simulink model "CONTROL_02"  (R2018b)
settings: Solver=FixedStepAuto  StartTime=0.0  StopTime=10  FixedStep=0.01  RelTol=1e-3
model workspace: external: MATLAB File D:\OneDrive\STUDY\RIC LAB\PROJECT 6DOF\CODE\CODE 6DOF\07_CONTROL\CONTROL_02\ROBOT_DataFile.m (data not in the file)
values from neighbouring files (symbols this model uses):
  k1 = [k11 k12 k13 k14 k15 k16]    [GA_CTC_01.m]
  k2 = [k21 k22 k23 k24 k25 k26]    [GA_CTC_01.m]
undefined symbols (not defined in the file or in its folder): smiData, X, Y, Z
libraries: sm_lib x35, nesl_utility x7
(part 1 of 14)
settings Model: Creator=TMP  LastModifiedBy=TMP
settings DataIOCC: SaveTime=off

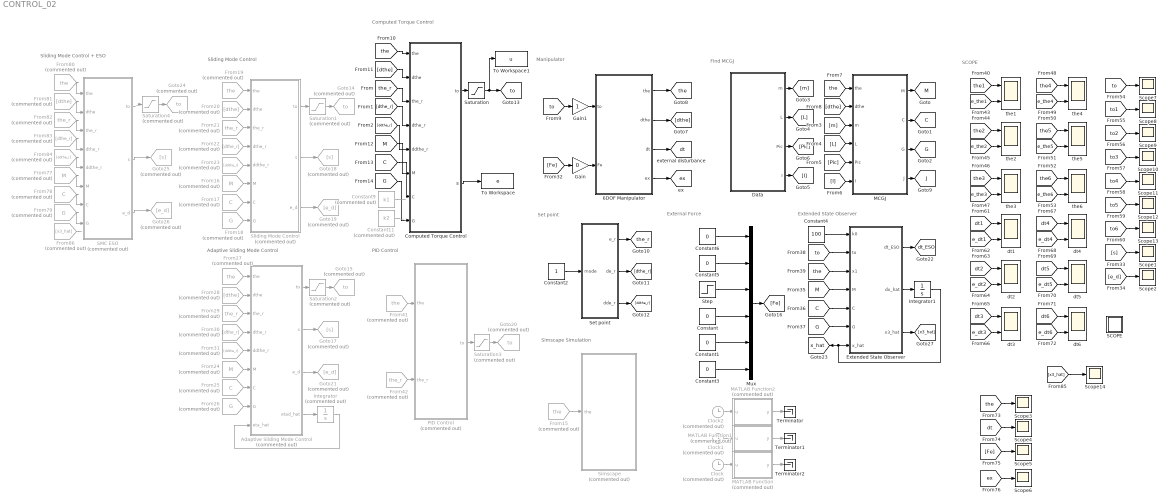
== system CONTROL_02 ==
  note: Extended State Observer
  note: SCOPE
  note: Set point
  note: Manipulator
  note: Simscape Simulation
  note: Find MCGJ
  note: Computed Torque Control
  note: Sliding Mode Control
  note: Adaptive Sliding Mode Control
  note: PID Control
  note: External Force
  note: Sliding Mode Control + ESO
  6DOF Manipulator : Subsystem
  Adaptive Sliding Mode Control : MATLAB Function  Commented=on  TreatAsAtomicUnit=on
  Clock : Clock  Commented=on
  Clock1 : Clock  Commented=on
  Clock2 : Clock  Commented=on
  Computed Torque Control : MATLAB Function  TreatAsAtomicUnit=on
  Constant{,1,3,5..6} (5 alike) : Constant  Value=0
  Constant11 : Constant  Commented=on  Value=k2
  Constant2 : Constant
  Constant4 : Constant  Value=100
  Constant9 : Constant  Commented=on  Value=k1
  Data : MATLAB Function  TreatAsAtomicUnit=on
  Extended State Observer : MATLAB Function  TreatAsAtomicUnit=on
  From{15,19,27,80} (4 alike) : From  Commented=on  GotoTag=the  TagVisibility=global
  From16 : From  Commented=on  GotoTag=M  TagVisibility=global
  From17 : From  Commented=on  GotoTag=C  TagVisibility=global
  From18 : From  Commented=on  GotoTag=G  TagVisibility=global
  From20 : From  Commented=on  GotoTag=dthe
  From21 : From  Commented=on  GotoTag=the_r  TagVisibility=global
  From22 : From  Commented=on  GotoTag=dthe_r
  From23 : From  Commented=on  GotoTag=ddthe_r
  From24 : From  Commented=on  GotoTag=M  TagVisibility=global
  From25 : From  Commented=on  GotoTag=C  TagVisibility=global
  From26 : From  Commented=on  GotoTag=G  TagVisibility=global
  From28 : From  Commented=on  GotoTag=dthe
  From29 : From  Commented=on  GotoTag=the_r  TagVisibility=global
  From30 : From  Commented=on  GotoTag=dthe_r
  From31 : From  Commented=on  GotoTag=ddthe_r
  From41 : From  Commented=on  GotoTag=the
  From42 : From  Commented=on  GotoTag=the_r
  From77 : From  Commented=on  GotoTag=M  TagVisibility=global
  From78 : From  Commented=on  GotoTag=C  TagVisibility=global
  From79 : From  Commented=on  GotoTag=G  TagVisibility=global
  From81 : From  Commented=on  GotoTag=dthe
  From82 : From  Commented=on  GotoTag=the_r  TagVisibility=global
  From83 : From  Commented=on  GotoTag=dthe_r
  From84 : From  Commented=on  GotoTag=ddthe_r
  From86 : From  Commented=on  GotoTag=x3_hat
  Gain : Gain  Gain=0
  Gain1 : Gain
  Goto{14..15,20,24} (4 alike) : Goto  Commented=on  GotoTag=to  TagVisibility=global
  Goto17 : Goto  Commented=on  GotoTag=s
  Goto18 : Goto  Commented=on  GotoTag=s
  Goto19 : Goto  Commented=on  GotoTag=e_d
  Goto21 : Goto  Commented=on  GotoTag=e_d
  Goto25 : Goto  Commented=on  GotoTag=s
  Goto26 : Goto  Commented=on  GotoTag=e_d
  Integrator : Integrator  Commented=on  InitialCondition=zeros(6)
  Integrator1 : Integrator  InitialCondition=zeros(18,1)
  MATLAB Function : MATLAB Function  Commented=on  TreatAsAtomicUnit=on
  MATLAB Function1 : MATLAB Function  Commented=on  TreatAsAtomicUnit=on
  MATLAB Function2 : MATLAB Function  Commented=on  TreatAsAtomicUnit=on
  MCGJ : MATLAB Function  TreatAsAtomicUnit=on
  Mux : Mux  Inputs=6
  PID Control : Subsystem  Commented=on
  SCOPE : Subsystem
  SMC ESO : MATLAB Function  Commented=on  TreatAsAtomicUnit=on
  Saturation : Saturate  UpperLimit=500  LowerLimit=-500
  Saturation1 : Saturate  Commented=on  UpperLimit=500  LowerLimit=-500
  Saturation2 : Saturate  Commented=on  UpperLimit=400  LowerLimit=-400
  Saturation3 : Saturate  Commented=on  UpperLimit=500  LowerLimit=-500
  Saturation4 : Saturate  Commented=on  UpperLimit=500  LowerLimit=-500
  Scope{1..14} (14 alike) : Scope
  Set point : Subsystem
  Simscape : Subsystem  Commented=on
  Sliding Mode Control : MATLAB Function  Commented=on  TreatAsAtomicUnit=on
  Step : Step  Time=5  After=20  SampleTime=0
  Terminator : Terminator
  Terminator1 : Terminator
  Terminator2 : Terminator
  To Workspace : ToWorkspace  VariableName=e  SampleTime=-1
  To Workspace1 : ToWorkspace  VariableName=u  SampleTime=-1
  dt{1..6} (6 alike) : Scope  NumInputPorts=2
  the{1..6} (6 alike) : Scope  NumInputPorts=2
  tag scope: C=global, G=global, J=global, M=global, dt=global, dt_ESO=global, ex=global, the=global, the_r=global, to=global, x_hat=global
  wires:
  [the_r] -> Computed Torque Control/3(the_r)
  Set point/3(dde_r) -> [ddthe_r]
  MCGJ/4(J) -> [J]
  [dthe] -> MCGJ/2(dthe)
  Set point/1(e_r) -> [the_r]
  [the] -> Computed Torque Control/1(the)
  [G] -> Computed Torque Control/8(G)
  [the] -> MCGJ/1(the)
  [dthe_r] -> Computed Torque Control/4(dthe_r)
  [C] -> Computed Torque Control/7(C)
  [M] -> Computed Torque Control/6(M)
  [ddthe_r] -> Computed Torque Control/5(ddthe_r)
  Constant2/1 -> Set point/1(mode)
  [m] -> MCGJ/3(m)
  Set point/2(de_r) -> [dthe_r]
  [dthe] -> Computed Torque Control/2(dthe)
  [L] -> MCGJ/4(L)
  MCGJ/3(G) -> [G]
  MCGJ/2(C) -> [C]
  [Pic] -> MCGJ/5(Pic)
  Saturation/1 -> To Workspace1/1, [to]
  [I] -> MCGJ/6(I)
  Computed Torque Control/1(to) -> Saturation/1
  MCGJ/1(M) -> [M]
  From16/1 -> Sliding Mode Control/6(M)
  From17/1 -> Sliding Mode Control/7(C)
  From18/1 -> Sliding Mode Control/8(G)
  From19/1 -> Sliding Mode Control/1(the)
  From20/1 -> Sliding Mode Control/2(dthe)
  From21/1 -> Sliding Mode Control/3(the_r)
  From22/1 -> Sliding Mode Control/4(dthe_r)
  From23/1 -> Sliding Mode Control/5(ddthe_r)
  Sliding Mode Control/1(to) -> Saturation1/1
  Saturation2/1 -> Goto15/1
  Adaptive Sliding Mode Control/1(to) -> Saturation2/1
  From31/1 -> Adaptive Sliding Mode Control/5(ddthe_r)
  From30/1 -> Adaptive Sliding Mode Control/4(dthe_r)
  From29/1 -> Adaptive Sliding Mode Control/3(the_r)
  From28/1 -> Adaptive Sliding Mode Control/2(dthe)
  From27/1 -> Adaptive Sliding Mode Control/1(the)
  From26/1 -> Adaptive Sliding Mode Control/8(G)
  From25/1 -> Adaptive Sliding Mode Control/7(C)
  From24/1 -> Adaptive Sliding Mode Control/6(M)
  Data/1(m) -> [m]
  Data/2(L) -> [L]
  Data/3(Pic) -> [Pic]
  Data/4(I) -> [I]
  6DOF Manipulator/2(dthe) -> [dthe]
  6DOF Manipulator/1(the) -> [the]
  From15/1 -> Simscape/1(the)
  Saturation1/1 -> Goto14/1
  [Fe] -> Gain/1
  Gain/1 -> 6DOF Manipulator/2(Fe)
  Adaptive Sliding Mode Control/2(s) -> Goto17/1
  Sliding Mode Control/2(s) -> Goto18/1
  Constant1/1 -> Mux/5
  Mux/1 -> [Fe]
  Constant3/1 -> Mux/6
  Constant/1 -> Mux/4
  PID Control/1(to) -> Saturation3/1
  From41/1 -> PID Control/1(the)
  From42/1 -> PID Control/2(the_r)
  Saturation3/1 -> Goto20/1
  6DOF Manipulator/3(dt) -> [dt]
  [to] -> Gain1/1
  Gain1/1 -> 6DOF Manipulator/1(to)
  Sliding Mode Control/3(e_d) -> Goto19/1
  Adaptive Sliding Mode Control/3(e_d) -> Goto21/1
  [the1] -> the1/1
  [e_the1] -> the1/2
  [e_the2] -> the2/2
  [the2] -> the2/1
  [the3] -> the3/1
  [e_the3] -> the3/2
  [e_the6] -> the6/2
  [the6] -> the6/1
  [the5] -> the5/1
  [e_the5] -> the5/2
  [e_the4] -> the4/2
  [the4] -> the4/1
  [to] -> Scope7/1
  [to1] -> Scope8/1
  [to2] -> Scope9/1
  [to5] -> Scope12/1
  [to4] -> Scope11/1
  [to3] -> Scope10/1
  [to6] -> Scope13/1
  [s] -> Scope1/1
  [e_d] -> Scope2/1
  Adaptive Sliding Mode Control/4(etad_hat) -> Integrator/1
  Integrator/1 -> Adaptive Sliding Mode Control/9(eta_hat)
  Extended State Observer/1(dt_ESO) -> [dt_ESO]
  Extended State Observer/2(dx_hat) -> Integrator1/1
  Constant4/1 -> Extended State Observer/1(k0)
  [to] -> Extended State Observer/2(to)
  [the] -> Extended State Observer/3(x1)
  [M] -> Extended State Observer/4(M)
  [C] -> Extended State Observer/5(C)
  [G] -> Extended State Observer/6(G)
  Integrator1/1 -> [x_hat], Extended State Observer/7(x_hat)
  [dt4] -> dt4/1
  [e_dt4] -> dt4/2
  [e_dt5] -> dt5/2
  [dt5] -> dt5/1
  [dt6] -> dt6/1
  [e_dt6] -> dt6/2
  [e_dt3] -> dt3/2
  [dt3] -> dt3/1
  [dt2] -> dt2/1
  [e_dt2] -> dt2/2
  [e_dt1] -> dt1/2
  [dt1] -> dt1/1
  [the] -> Scope3/1
  [dt] -> Scope4/1
  MATLAB Function1/1(y) -> Terminator1/1
  Clock1/1 -> MATLAB Function1/1(u)
  Clock/1 -> MATLAB Function/1(u)
  MATLAB Function/1(y) -> Terminator2/1
  Clock2/1 -> MATLAB Function2/1(u)
  MATLAB Function2/1(y) -> Terminator/1
  Step/1 -> Mux/3
  Constant6/1 -> Mux/1
  Constant5/1 -> Mux/2
  [Fe] -> Scope5/1
  6DOF Manipulator/4(ex) -> [ex]
  [ex] -> Scope6/1
  Computed Torque Control/2(E) -> To Workspace/1
  Constant9/1 -> ?
  Constant11/1 -> ?
  SMC ESO/3(e_d) -> Goto26/1
  SMC ESO/2(s) -> Goto25/1
  Saturation4/1 -> Goto24/1
  SMC ESO/1(to) -> Saturation4/1
  From84/1 -> SMC ESO/5(ddthe_r)
  From83/1 -> SMC ESO/4(dthe_r)
  From82/1 -> SMC ESO/3(the_r)
  From81/1 -> SMC ESO/2(dthe)
  From80/1 -> SMC ESO/1(the)
  From79/1 -> SMC ESO/8(G)
  From78/1 -> SMC ESO/7(C)
  From77/1 -> SMC ESO/6(M)
  From86/1 -> ?
  Extended State Observer/3(x3_hat) -> [x3_hat]
  [x3_hat] -> Scope14/1

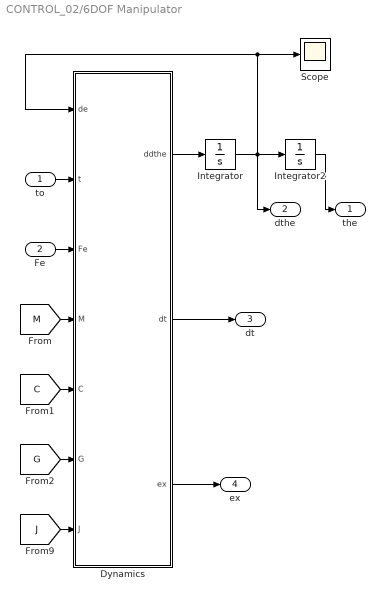
== system CONTROL_02/6DOF Manipulator ==
  to : Inport
  Fe : Inport  Port=2
  Dynamics : MATLAB Function  TreatAsAtomicUnit=on
  Integrator : Integrator  InitialCondition=[0;0;0;0;0;0]  UpperSaturationLimit=pi  LowerSaturationLimit=-pi
  Integrator2 : Integrator  InitialCondition=[0;0;0;0;0;0]  UpperSaturationLimit=[170;135;166;190;120;360]*pi/180  LowerSaturationLimit=-[170;100;119;190;120;360]*pi/180
  Scope : Scope
  the : Outport
  dthe : Outport  Port=2
  dt : Outport  Port=3
  ex : Outport  Port=4
  wires:
  Integrator2/1 -> the/1
  Dynamics/1(ddthe) -> Integrator/1
  [C] -> Dynamics/5(C)
  [J] -> Dynamics/7(J)
  Integrator/1 -> Integrator2/1, Scope/1, Dynamics/1(de), dthe/1
  [M] -> Dynamics/4(M)
  [G] -> Dynamics/6(G)
  to/1 -> Dynamics/2(t)
  Dynamics/2(dt) -> dt/1
  Fe/1 -> Dynamics/3(Fe)
  Dynamics/3(ex) -> ex/1

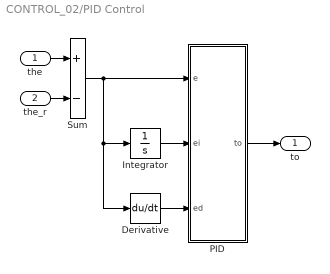
== system CONTROL_02/PID Control ==
  the : Inport
  the_r : Inport  Port=2
  Derivative : Derivative
  Integrator : Integrator
  PID : MATLAB Function  TreatAsAtomicUnit=on
  Sum : Sum  Inputs=+-
  to : Outport
  wires:
  Sum/1 -> Derivative/1, Integrator/1, PID/1(e)
  the/1 -> Sum/1
  the_r/1 -> Sum/2
  PID/1(to) -> to/1
  Derivative/1 -> PID/3(ed)
  Integrator/1 -> PID/2(ei)

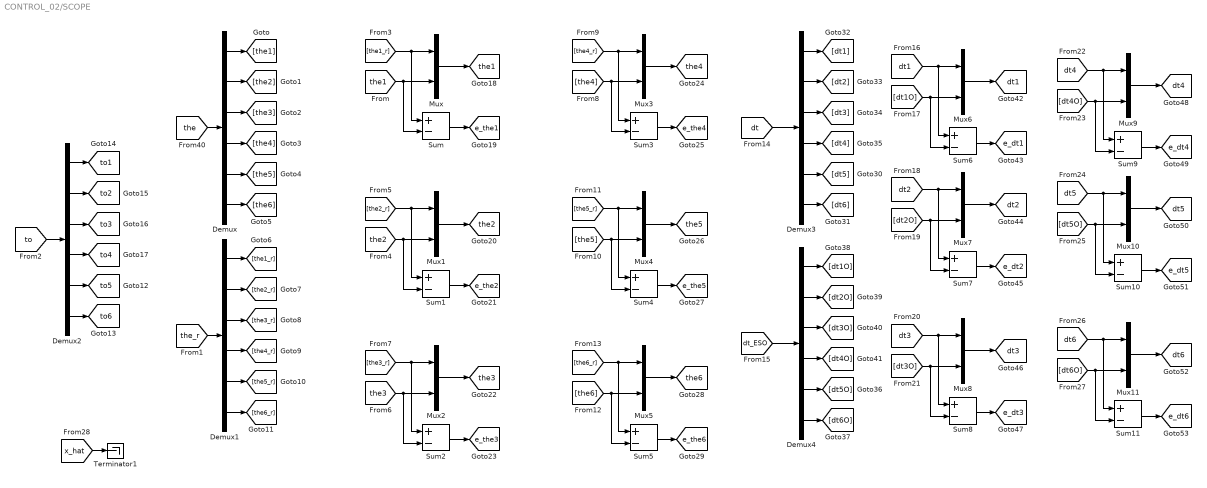
== system CONTROL_02/SCOPE ==
  Demux{,1..4} (5 alike) : Demux  Outputs=6
  Mux{,1..11} (12 alike) : Mux  Inputs=2
  Sum{,1..11} (12 alike) : Sum  Inputs=+-
  Terminator1 : Terminator
  tag scope: dt1=global, dt2=global, dt3=global, dt4=global, dt5=global, dt6=global, e_dt1=global, e_dt2=global, e_dt3=global, e_dt4=global, e_dt5=global, e_dt6=global, e_the1=global, e_the2=global, e_the3=global, e_the4=global, e_the5=global, e_the6=global, the1=global, the2=global, the3=global, the4=global, the5=global, the6=global, to1=global, to2=global, to3=global, to4=global, to5=global, to6=global
  wires:
  Demux/4 -> [the4]
  Demux/6 -> [the6]
  [the] -> Demux/1
  Demux/1 -> [the1]
  Demux/5 -> [the5]
  Demux/2 -> [the2]
  Demux/3 -> [the3]
  Demux1/1 -> [the1_r]
  Demux1/4 -> [the4_r]
  [the_r] -> Demux1/1
  Demux1/5 -> [the5_r]
  Demux1/2 -> [the2_r]
  Demux1/3 -> [the3_r]
  Demux1/6 -> [the6_r]
  Demux2/6 -> [to6]
  Demux2/3 -> [to3]
  Demux2/2 -> [to2]
  Demux2/4 -> [to4]
  Demux2/5 -> [to5]
  [to] -> Demux2/1
  Demux2/1 -> [to1]
  [the1_r] -> Sum/1, Mux/1
  [the1] -> Mux/2, Sum/2
  Mux/1 -> [the1]
  Sum/1 -> [e_the1]
  Sum1/1 -> [e_the2]
  Mux1/1 -> [the2]
  [the2] -> Sum1/2, Mux1/2
  [the2_r] -> Mux1/1, Sum1/1
  [the3_r] -> Sum2/1, Mux2/1
  [the3] -> Mux2/2, Sum2/2
  Mux2/1 -> [the3]
  Sum2/1 -> [e_the3]
  Sum5/1 -> [e_the6]
  Mux5/1 -> [the6]
  [the6] -> Sum5/2, Mux5/2
  [the6_r] -> Mux5/1, Sum5/1
  [the5_r] -> Sum4/1, Mux4/1
  [the5] -> Mux4/2, Sum4/2
  Mux4/1 -> [the5]
  Sum4/1 -> [e_the5]
  Sum3/1 -> [e_the4]
  Mux3/1 -> [the4]
  [the4] -> Sum3/2, Mux3/2
  [the4_r] -> Mux3/1, Sum3/1
  Demux3/1 -> [dt1]
  Demux3/5 -> [dt5]
  Demux3/4 -> [dt4]
  Demux3/2 -> [dt2]
  Demux3/3 -> [dt3]
  Demux3/6 -> [dt6]
  [dt] -> Demux3/1
  [dt_ESO] -> Demux4/1
  Demux4/6 -> [dt6O]
  Demux4/3 -> [dt3O]
  Demux4/2 -> [dt2O]
  Demux4/4 -> [dt4O]
  Demux4/5 -> [dt5O]
  Demux4/1 -> [dt1O]
  Sum6/1 -> [e_dt1]
  Mux6/1 -> [dt1]
  [dt1O] -> Sum6/2, Mux6/2
  [dt1] -> Mux6/1, Sum6/1
  [dt2] -> Sum7/1, Mux7/1
  [dt2O] -> Mux7/2, Sum7/2
  Mux7/1 -> [dt2]
  Sum7/1 -> [e_dt2]
  Sum8/1 -> [e_dt3]
  Mux8/1 -> [dt3]
  [dt3O] -> Sum8/2, Mux8/2
  [dt3] -> Mux8/1, Sum8/1
  [dt6] -> Sum11/1, Mux11/1
  [dt6O] -> Mux11/2, Sum11/2
  Mux11/1 -> [dt6]
  Sum11/1 -> [e_dt6]
  Sum10/1 -> [e_dt5]
  Mux10/1 -> [dt5]
  [dt5O] -> Sum10/2, Mux10/2
  [dt5] -> Mux10/1, Sum10/1
  [dt4] -> Sum9/1, Mux9/1
  [dt4O] -> Mux9/2, Sum9/2
  Mux9/1 -> [dt4]
  Sum9/1 -> [e_dt4]
  [x_hat] -> Terminator1/1

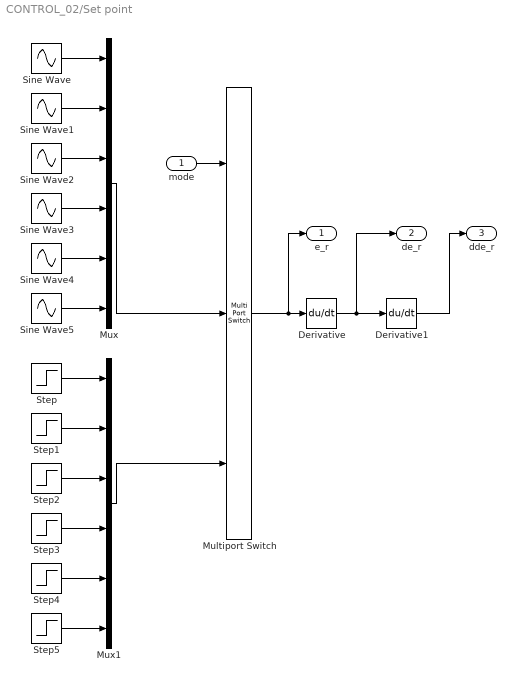
== system CONTROL_02/Set point ==
  mode : Inport
  Derivative : Derivative
  Derivative1 : Derivative
  Multiport Switch : MultiPortSwitch  Inputs=2
  Mux : Mux  Inputs=6
  Mux1 : Mux  Inputs=6
  Sine Wave{,1..5} (6 alike) : Sin  Amplitude=pi/6  Frequency=2*pi*0.1  SampleTime=0
  Step{,1..5} (6 alike) : Step  After=0  SampleTime=0
  e_r : Outport
  de_r : Outport  Port=2
  dde_r : Outport  Port=3
  wires:
  Sine Wave/1 -> Mux/1
  Sine Wave1/1 -> Mux/2
  Sine Wave2/1 -> Mux/3
  Sine Wave3/1 -> Mux/4
  Sine Wave4/1 -> Mux/5
  Sine Wave5/1 -> Mux/6
  Mux/1 -> Multiport Switch/2
  Mux1/1 -> Multiport Switch/3
  Step2/1 -> Mux1/3
  Step5/1 -> Mux1/6
  Step1/1 -> Mux1/2
  Step3/1 -> Mux1/4
  Step/1 -> Mux1/1
  Step4/1 -> Mux1/5
  Multiport Switch/1 -> e_r/1, Derivative/1
  Derivative/1 -> de_r/1, Derivative1/1
  Derivative1/1 -> dde_r/1
  mode/1 -> Multiport Switch/1

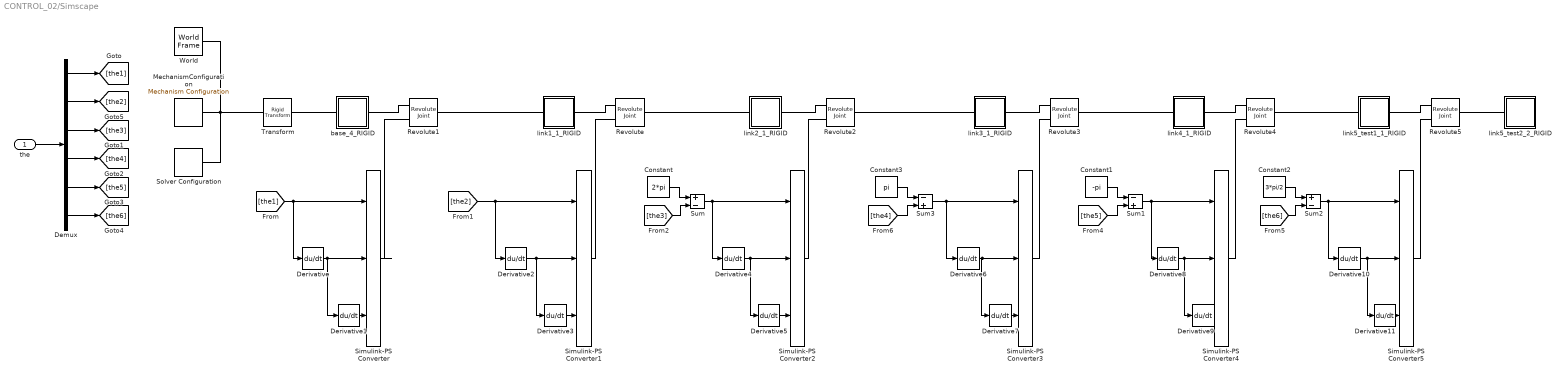
== system CONTROL_02/Simscape ==
  the : Inport
  Constant : Constant  Value=2*pi
  Constant1 : Constant  Value=-pi
  Constant2 : Constant  Value=3*pi/2
  Constant3 : Constant  Value=pi
  Demux : Demux  Outputs=6
  Derivative{,1..11} (12 alike) : Derivative
  MechanismConfiguration : sm_lib/Utilities/Mechanism Configuration  UniformGravity=Constant  GravityVector=[0 -9.80665 0]  GravityUnits=m/s^2  LinearizationDelta=0.001
  Revolute : sm_lib/Joints/Revolute Joint  SenseConstraintForce=off  SenseConstraintForceX=off  SenseConstraintForceY=off  SenseConstraintForceZ=off  SenseConstraintTorque=off  SenseConstraintTorqueX=off  SenseConstraintTorqueY=off  SenseConstraintTorqueZ=off  SenseTotalForce=off  SenseTotalForceX=off  SenseTotalForceY=off  SenseTotalForceZ=off  SenseTotalTorque=off  SenseTotalTorqueX=off  SenseTotalTorqueY=off  SenseTotalTorqueZ=off  CompositeWrenchDir=FollowerOnBase  CompositeWrenchFrame=BaseFrame  EquilibriumPosition=0  EquilibriumPositionUnits=rad  SpringStiffness=0  SpringStiffnessUnits=N*m/rad  DampingCoefficient=0  DampingCoefficientUnits=N*m/(rad/s)  TorqueActuationMode=ComputedTorque  MotionActuationMode=InputMotion  SensePosition=off  SenseVelocity=off  SenseAcceleration=off  SenseTorqueForce=off  PositionTargetSpecify=on  PositionTargetPriority=Low  PositionTargetValue=smiData.RevoluteJoint(1).Rz.Pos  PositionTargetValueUnits=deg  VelocityTargetSpecify=off  VelocityTargetPriority=High  VelocityTargetValue=0  VelocityTargetValueUnits=deg/s
  Revolute1 : sm_lib/Joints/Revolute Joint  SenseConstraintForce=off  SenseConstraintForceX=off  SenseConstraintForceY=off  SenseConstraintForceZ=off  SenseConstraintTorque=off  SenseConstraintTorqueX=off  SenseConstraintTorqueY=off  SenseConstraintTorqueZ=off  SenseTotalForce=off  SenseTotalForceX=off  SenseTotalForceY=off  SenseTotalForceZ=off  SenseTotalTorque=off  SenseTotalTorqueX=off  SenseTotalTorqueY=off  SenseTotalTorqueZ=off  CompositeWrenchDir=FollowerOnBase  CompositeWrenchFrame=BaseFrame  EquilibriumPosition=0  EquilibriumPositionUnits=rad  SpringStiffness=0  SpringStiffnessUnits=N*m/rad  DampingCoefficient=0  DampingCoefficientUnits=N*m/(rad/s)  TorqueActuationMode=ComputedTorque  MotionActuationMode=InputMotion  SensePosition=off  SenseVelocity=off  SenseAcceleration=off  SenseTorqueForce=off  PositionTargetSpecify=on  PositionTargetPriority=Low  PositionTargetValue=smiData.RevoluteJoint(2).Rz.Pos  PositionTargetValueUnits=deg  VelocityTargetSpecify=off  VelocityTargetPriority=High  VelocityTargetValue=0  VelocityTargetValueUnits=deg/s
  Revolute2 : sm_lib/Joints/Revolute Joint  SenseConstraintForce=off  SenseConstraintForceX=off  SenseConstraintForceY=off  SenseConstraintForceZ=off  SenseConstraintTorque=off  SenseConstraintTorqueX=off  SenseConstraintTorqueY=off  SenseConstraintTorqueZ=off  SenseTotalForce=off  SenseTotalForceX=off  SenseTotalForceY=off  SenseTotalForceZ=off  SenseTotalTorque=off  SenseTotalTorqueX=off  SenseTotalTorqueY=off  SenseTotalTorqueZ=off  CompositeWrenchDir=FollowerOnBase  CompositeWrenchFrame=BaseFrame  EquilibriumPosition=0  EquilibriumPositionUnits=rad  SpringStiffness=0  SpringStiffnessUnits=N*m/rad  DampingCoefficient=0  DampingCoefficientUnits=N*m/(rad/s)  TorqueActuationMode=ComputedTorque  MotionActuationMode=InputMotion  SensePosition=off  SenseVelocity=off  SenseAcceleration=off  SenseTorqueForce=off  PositionTargetSpecify=on  PositionTargetPriority=Low  PositionTargetValue=smiData.RevoluteJoint(3).Rz.Pos  PositionTargetValueUnits=deg  VelocityTargetSpecify=off  VelocityTargetPriority=High  VelocityTargetValue=0  VelocityTargetValueUnits=deg/s
  Revolute3 : sm_lib/Joints/Revolute Joint  SenseConstraintForce=off  SenseConstraintForceX=off  SenseConstraintForceY=off  SenseConstraintForceZ=off  SenseConstraintTorque=off  SenseConstraintTorqueX=off  SenseConstraintTorqueY=off  SenseConstraintTorqueZ=off  SenseTotalForce=off  SenseTotalForceX=off  SenseTotalForceY=off  SenseTotalForceZ=off  SenseTotalTorque=off  SenseTotalTorqueX=off  SenseTotalTorqueY=off  SenseTotalTorqueZ=off  CompositeWrenchDir=FollowerOnBase  CompositeWrenchFrame=BaseFrame  EquilibriumPosition=0  EquilibriumPositionUnits=rad  SpringStiffness=0  SpringStiffnessUnits=N*m/rad  DampingCoefficient=0  DampingCoefficientUnits=N*m/(rad/s)  TorqueActuationMode=ComputedTorque  MotionActuationMode=InputMotion  SensePosition=off  SenseVelocity=off  SenseAcceleration=off  SenseTorqueForce=off  PositionTargetSpecify=on  PositionTargetPriority=Low  PositionTargetValue=smiData.RevoluteJoint(4).Rz.Pos  PositionTargetValueUnits=deg  VelocityTargetSpecify=off  VelocityTargetPriority=High  VelocityTargetValue=0  VelocityTargetValueUnits=deg/s
  Revolute4 : sm_lib/Joints/Revolute Joint  SenseConstraintForce=off  SenseConstraintForceX=off  SenseConstraintForceY=off  SenseConstraintForceZ=off  SenseConstraintTorque=off  SenseConstraintTorqueX=off  SenseConstraintTorqueY=off  SenseConstraintTorqueZ=off  SenseTotalForce=off  SenseTotalForceX=off  SenseTotalForceY=off  SenseTotalForceZ=off  SenseTotalTorque=off  SenseTotalTorqueX=off  SenseTotalTorqueY=off  SenseTotalTorqueZ=off  CompositeWrenchDir=FollowerOnBase  CompositeWrenchFrame=BaseFrame  EquilibriumPosition=0  EquilibriumPositionUnits=rad  SpringStiffness=0  SpringStiffnessUnits=N*m/rad  DampingCoefficient=0  DampingCoefficientUnits=N*m/(rad/s)  TorqueActuationMode=ComputedTorque  MotionActuationMode=InputMotion  SensePosition=off  SenseVelocity=off  SenseAcceleration=off  SenseTorqueForce=off  PositionTargetSpecify=on  PositionTargetPriority=Low  PositionTargetValue=smiData.RevoluteJoint(5).Rz.Pos  PositionTargetValueUnits=deg  VelocityTargetSpecify=off  VelocityTargetPriority=High  VelocityTargetValue=0  VelocityTargetValueUnits=deg/s
  Revolute5 : sm_lib/Joints/Revolute Joint  SenseConstraintForce=off  SenseConstraintForceX=off  SenseConstraintForceY=off  SenseConstraintForceZ=off  SenseConstraintTorque=off  SenseConstraintTorqueX=off  SenseConstraintTorqueY=off  SenseConstraintTorqueZ=off  SenseTotalForce=off  SenseTotalForceX=off  SenseTotalForceY=off  SenseTotalForceZ=off  SenseTotalTorque=off  SenseTotalTorqueX=off  SenseTotalTorqueY=off  SenseTotalTorqueZ=off  CompositeWrenchDir=FollowerOnBase  CompositeWrenchFrame=BaseFrame  EquilibriumPosition=0  EquilibriumPositionUnits=rad  SpringStiffness=0  SpringStiffnessUnits=N*m/rad  DampingCoefficient=0  DampingCoefficientUnits=N*m/(rad/s)  TorqueActuationMode=ComputedTorque  MotionActuationMode=InputMotion  SensePosition=off  SenseVelocity=off  SenseAcceleration=off  SenseTorqueForce=off  PositionTargetSpecify=on  PositionTargetPriority=Low  PositionTargetValue=smiData.RevoluteJoint(6).Rz.Pos  PositionTargetValueUnits=deg  VelocityTargetSpecify=off  VelocityTargetPriority=High  VelocityTargetValue=0  VelocityTargetValueUnits=deg/s
  Simulink-PS Converter{,1..5} (6 alike) : nesl_utility/Simulink-PS Converter  PhysicalDomain=network_engine_domain  SubClassName=ps_input  LeftPortType=input  RightPortType=output  PseudoPeriodic=off  Frequencies=[]  NoiseDistribution=none  NoiseParameters=[]  Unit=1  AffineConversion=off  FilteringAndDerivatives=provide  SimscapeFilterOrder=1  InputFilterTimeConstant=0.001  UdotUserProvided=2
  Solver Configuration : nesl_utility/Solver Configuration  PhysicalDomain=network_engine_domain  SubClassName=solver  LeftPortType=input  RightPortType=generic  Tones=[]  Harmonics=[]  SimulateNoise=off  Profile=off  UseLocalSampling=off  EnableSwitchedLinearOptims=on  FrequencyDomain=off  UseCCode=off  RelTol=0.001  AbsTol=1e-06  MinStep=1e-09  ToWorkspace=off  RevertToSquareIcSolve=off  NumHomotopyIterations=100  PhasorMode=off  PhasorModeNumHarmonics=1  DoDC=off  ResidualTolerance=1e-09  UseLocalSolver=off  LocalSolverChoice=NE_BACKWARD_EULER_ADVANCER  LocalSolverSampleTime=0.001  DoFixedCost=off  MaxNonlinIter=3  MaxModeIter=2  LinearAlgebra=auto  EquationFormulation=NE_TIME_EF  DelaysMemoryBudget=1024  AutomaticFiltering=on  FilteringTimeConstant=0.001  PartitionStorageMethod=AS_NEEDED  PartitionMemoryBudget=1024
  Sum : Sum  Inputs=+-
  Sum1 : Sum  Inputs=-+
  Sum2 : Sum  Inputs=+-
  Sum3 : Sum  Inputs=-+
  Transform : sm_lib/Frames and Transforms/Rigid Transform  TranslationMethod=Cartesian  TranslationStandardOffset=0  TranslationLengthUnit=m  TranslationStandardAxis=+Z  TranslationCartesianOffset=smiData.RigidTransform(13).translation  TranslationROffset=0  TranslationROffsetUnits=m  TranslationZOffset=0  TranslationZOffsetUnits=m  TranslationThetaOffset=0  TranslationThetaOffsetUnits=deg  RotationMethod=ArbitraryAxis  RotationAngleUnits=rad  RotationStandardAxis=+Z  RotationAngle=smiData.RigidTransform(13).angle  RotationArbitraryAxis=smiData.RigidTransform(13).axis  FollAlignAxisA=+X  BaseAlignAxisA=+Y  FollAlignAxisB=+Y  BaseAlignAxisB=+Z  RotationSequenceAxes=FollowerAxes  RotationSequence=XYX  RotationSequenceAngles=[0 0 0]  RotationSequenceAnglesUnits=deg  RotationMatrix=[1 0 0; 0 1 0; 0 0 1]
  World : sm_lib/Frames and Transforms/World Frame
  base_4_RIGID : Subsystem
  link1_1_RIGID : Subsystem
  link2_1_RIGID : Subsystem
  link3_1_RIGID : Subsystem
  link4_1_RIGID : Subsystem
  link5_test1_1_RIGID : Subsystem
  link5_test2_2_RIGID : Subsystem
  wires:
  Derivative2/1 -> Derivative3/1, Simulink-PS Converter1/2
  [the2] -> Derivative2/1, Simulink-PS Converter1/1
  Derivative11/1 -> Simulink-PS Converter5/3
  [the6] -> Sum2/2
  Demux/5 -> [the5]
  Sum3/1 -> Derivative6/1, Simulink-PS Converter3/1
  [the3] -> Sum/2
  Derivative4/1 -> Derivative5/1, Simulink-PS Converter2/2
  Derivative7/1 -> Simulink-PS Converter3/3
  Demux/1 -> [the1]
  Sum/1 -> Simulink-PS Converter2/1, Derivative4/1
  Sum1/1 -> Derivative8/1, Simulink-PS Converter4/1
  Derivative8/1 -> Derivative9/1, Simulink-PS Converter4/2
  Demux/2 -> [the2]
  Demux/3 -> [the3]
  Derivative10/1 -> Simulink-PS Converter5/2, Derivative11/1
  Demux/4 -> [the4]
  the/1 -> Demux/1
  [the5] -> Sum1/2
  Demux/6 -> [the6]
  Sum2/1 -> Derivative10/1, Simulink-PS Converter5/1
  [the1] -> Derivative/1, Simulink-PS Converter/1
  Derivative6/1 -> Derivative7/1, Simulink-PS Converter3/2
  Constant2/1 -> Sum2/1
  Derivative/1 -> Derivative1/1, Simulink-PS Converter/2
  Derivative5/1 -> Simulink-PS Converter2/3
  Derivative1/1 -> Simulink-PS Converter/3
  Constant1/1 -> Sum1/1
  Derivative9/1 -> Simulink-PS Converter4/3
  Derivative3/1 -> Simulink-PS Converter1/3
  Constant/1 -> Sum/1
  Constant3/1 -> Sum3/1
  [the4] -> Sum3/2
  connections:
  Simulink-PS Converter/RConn1 -- Revolute1/LConn2
  Revolute/RConn1 -- link2_1_RIGID/LConn1
  Revolute3/RConn1 -- link4_1_RIGID/LConn1
  Revolute1/RConn1 -- link1_1_RIGID/LConn1
  Revolute4/LConn2 -- Simulink-PS Converter4/RConn1
  Revolute2/LConn2 -- Simulink-PS Converter2/RConn1
  Transform/RConn1 -- base_4_RIGID/LConn1
  Revolute1/LConn1 -- base_4_RIGID/RConn1
  Revolute/LConn1 -- link1_1_RIGID/RConn1
  Revolute/LConn2 -- Simulink-PS Converter1/RConn1
  Revolute4/RConn1 -- link5_test1_1_RIGID/LConn1
  Revolute5/LConn1 -- link5_test1_1_RIGID/RConn1
  Revolute3/LConn2 -- Simulink-PS Converter3/RConn1
  Revolute5/RConn1 -- link5_test2_2_RIGID/LConn1
  Transform/LConn1 -- MechanismConfiguration/RConn1 -- Solver Configuration/RConn1 -- World/RConn1
  Revolute5/LConn2 -- Simulink-PS Converter5/RConn1
  Revolute2/RConn1 -- link3_1_RIGID/LConn1
  Revolute2/LConn1 -- link2_1_RIGID/RConn1
  Revolute3/LConn1 -- link3_1_RIGID/RConn1
  Revolute4/LConn1 -- link4_1_RIGID/RConn1

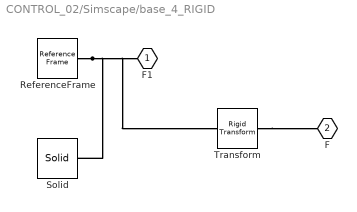
== system CONTROL_02/Simscape/base_4_RIGID ==
  ReferenceFrame : sm_lib/Frames and Transforms/Reference Frame
  Solid : sm_lib/Body Elements/Solid  InertiaType=Custom  Mass=smiData.Solid(1).mass  MassUnits=kg  CenterOfMass=smiData.Solid(1).CoM  CenterOfMassUnits=m  MomentsOfInertia=smiData.Solid(1).MoI  MomentsOfInertiaUnits=kg*m^2  ProductsOfInertia=smiData.Solid(1).PoI  ProductsOfInertiaUnits=kg*m^2  BasedOnType=Density  Density=1000  DensityUnits=kg/m^3  DoExposeReferenceFrame=on  SerializedFrames=<Frames/>  GraphicType=FromGeometry  MarkerShape=Sphere  MarkerSize=10  GraphicVisPropType=SimpleVisualProperties  GraphicDiffuseColor=smiData.Solid(1).color  GraphicSpecularColor=[0.5 0.5 0.5 1.0]  GraphicAmbientColor=[0.15 0.15 0.15 1.0]  GraphicEmissiveColor=[0.0 0.0 0.0 1.0]  GraphicShininess=75  GraphicOpacity=smiData.Solid(1).opacity  GeometryShape=FromFile  RectangleSize=[1 1]  RectangleSizeUnits=m  BrickDimensions=[1 1 1]  BrickDimensionUnits=m  CylinderRadius=1  CylinderRadiusUnits=m  CylinderLength=1  CylinderLengthUnits=m  SphereRadius=1  SphereRadiusUnits=m  EllipsoidRadii=[1 1 1]  EllipsoidRadiiUnits=m  ExtrusionCrossSection=[1 1; -1 1; -1 -1; 1 -1]  ExtrusionCrossSectionUnits=m  ExtrusionLength=1  ExtrusionLengthUnits=m  PolygonNumSides=3  PolygonOuterRadius=1  PolygonOuterRadiusUnits=m  ExtGeomFileType=STEP  ExtGeomFileName=base_Default_sldprt.STEP  ExtGeomFileUnits=m  RevolutionCrossSection=[1 1; 1 -1; 2 -1; 2 1]  RevolutionCrossSectionUnits=m  RevolutionExtent=Full  RevolutionAngle=180  RevolutionAngleUnits=deg
  Transform : sm_lib/Frames and Transforms/Rigid Transform  TranslationMethod=Cartesian  TranslationStandardOffset=0  TranslationLengthUnit=m  TranslationStandardAxis=+Z  TranslationCartesianOffset=smiData.RigidTransform(3).translation  TranslationROffset=0  TranslationROffsetUnits=m  TranslationZOffset=0  TranslationZOffsetUnits=m  TranslationThetaOffset=0  TranslationThetaOffsetUnits=deg  RotationMethod=ArbitraryAxis  RotationAngleUnits=rad  RotationStandardAxis=+Z  RotationAngle=smiData.RigidTransform(3).angle  RotationArbitraryAxis=smiData.RigidTransform(3).axis  FollAlignAxisA=+X  BaseAlignAxisA=+Y  FollAlignAxisB=+Y  BaseAlignAxisB=+Z  RotationSequenceAxes=FollowerAxes  RotationSequence=XYX  RotationSequenceAngles=[0 0 0]  RotationSequenceAnglesUnits=deg  RotationMatrix=[1 0 0; 0 1 0; 0 0 1]
  F1 : PMIOPort  Side=Left
  F : PMIOPort  Port=2  Side=Right
  connections:
  Solid/RConn1 -- ReferenceFrame/RConn1 -- Transform/LConn1 -- F1/RConn1
  Transform/RConn1 -- F/RConn1

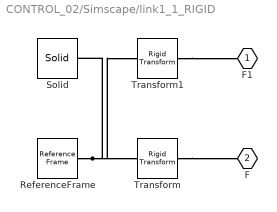
== system CONTROL_02/Simscape/link1_1_RIGID ==
  ReferenceFrame : sm_lib/Frames and Transforms/Reference Frame
  Solid : sm_lib/Body Elements/Solid  InertiaType=Custom  Mass=smiData.Solid(2).mass  MassUnits=kg  CenterOfMass=smiData.Solid(2).CoM  CenterOfMassUnits=m  MomentsOfInertia=smiData.Solid(2).MoI  MomentsOfInertiaUnits=kg*m^2  ProductsOfInertia=smiData.Solid(2).PoI  ProductsOfInertiaUnits=kg*m^2  BasedOnType=Density  Density=1000  DensityUnits=kg/m^3  DoExposeReferenceFrame=on  SerializedFrames=<Frames/>  GraphicType=FromGeometry  MarkerShape=Sphere  MarkerSize=10  GraphicVisPropType=SimpleVisualProperties  GraphicDiffuseColor=smiData.Solid(2).color  GraphicSpecularColor=[0.5 0.5 0.5 1.0]  GraphicAmbientColor=[0.15 0.15 0.15 1.0]  GraphicEmissiveColor=[0.0 0.0 0.0 1.0]  GraphicShininess=75  GraphicOpacity=smiData.Solid(2).opacity  GeometryShape=FromFile  RectangleSize=[1 1]  RectangleSizeUnits=m  BrickDimensions=[1 1 1]  BrickDimensionUnits=m  CylinderRadius=1  CylinderRadiusUnits=m  CylinderLength=1  CylinderLengthUnits=m  SphereRadius=1  SphereRadiusUnits=m  EllipsoidRadii=[1 1 1]  EllipsoidRadiiUnits=m  ExtrusionCrossSection=[1 1; -1 1; -1 -1; 1 -1]  ExtrusionCrossSectionUnits=m  ExtrusionLength=1  ExtrusionLengthUnits=m  PolygonNumSides=3  PolygonOuterRadius=1  PolygonOuterRadiusUnits=m  ExtGeomFileType=STEP  ExtGeomFileName=link1_Default_sldprt.STEP  ExtGeomFileUnits=m  RevolutionCrossSection=[1 1; 1 -1; 2 -1; 2 1]  RevolutionCrossSectionUnits=m  RevolutionExtent=Full  RevolutionAngle=180  RevolutionAngleUnits=deg
  Transform : sm_lib/Frames and Transforms/Rigid Transform  TranslationMethod=Cartesian  TranslationStandardOffset=0  TranslationLengthUnit=m  TranslationStandardAxis=+Z  TranslationCartesianOffset=smiData.RigidTransform(1).translation  TranslationROffset=0  TranslationROffsetUnits=m  TranslationZOffset=0  TranslationZOffsetUnits=m  TranslationThetaOffset=0  TranslationThetaOffsetUnits=deg  RotationMethod=ArbitraryAxis  RotationAngleUnits=rad  RotationStandardAxis=+Z  RotationAngle=smiData.RigidTransform(1).angle  RotationArbitraryAxis=smiData.RigidTransform(1).axis  FollAlignAxisA=+X  BaseAlignAxisA=+Y  FollAlignAxisB=+Y  BaseAlignAxisB=+Z  RotationSequenceAxes=FollowerAxes  RotationSequence=XYX  RotationSequenceAngles=[0 0 0]  RotationSequenceAnglesUnits=deg  RotationMatrix=[1 0 0; 0 1 0; 0 0 1]
  Transform1 : sm_lib/Frames and Transforms/Rigid Transform  TranslationMethod=Cartesian  TranslationStandardOffset=0  TranslationLengthUnit=m  TranslationStandardAxis=+Z  TranslationCartesianOffset=smiData.RigidTransform(4).translation  TranslationROffset=0  TranslationROffsetUnits=m  TranslationZOffset=0  TranslationZOffsetUnits=m  TranslationThetaOffset=0  TranslationThetaOffsetUnits=deg  RotationMethod=ArbitraryAxis  RotationAngleUnits=rad  RotationStandardAxis=+Z  RotationAngle=smiData.RigidTransform(4).angle  RotationArbitraryAxis=smiData.RigidTransform(4).axis  FollAlignAxisA=+X  BaseAlignAxisA=+Y  FollAlignAxisB=+Y  BaseAlignAxisB=+Z  RotationSequenceAxes=FollowerAxes  RotationSequence=XYX  RotationSequenceAngles=[0 0 0]  RotationSequenceAnglesUnits=deg  RotationMatrix=[1 0 0; 0 1 0; 0 0 1]
  F1 : PMIOPort  Side=Left
  F : PMIOPort  Port=2  Side=Right
  connections:
  Solid/RConn1 -- ReferenceFrame/RConn1 -- Transform/LConn1 -- Transform1/LConn1
  Transform/RConn1 -- F/RConn1
  Transform1/RConn1 -- F1/RConn1

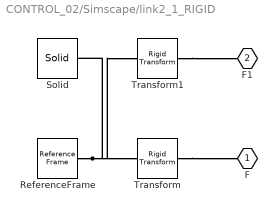
== system CONTROL_02/Simscape/link2_1_RIGID ==
  ReferenceFrame : sm_lib/Frames and Transforms/Reference Frame
  Solid : sm_lib/Body Elements/Solid  InertiaType=Custom  Mass=smiData.Solid(5).mass  MassUnits=kg  CenterOfMass=smiData.Solid(5).CoM  CenterOfMassUnits=m  MomentsOfInertia=smiData.Solid(5).MoI  MomentsOfInertiaUnits=kg*m^2  ProductsOfInertia=smiData.Solid(5).PoI  ProductsOfInertiaUnits=kg*m^2  BasedOnType=Density  Density=1000  DensityUnits=kg/m^3  DoExposeReferenceFrame=on  SerializedFrames=<Frames/>  GraphicType=FromGeometry  MarkerShape=Sphere  MarkerSize=10  GraphicVisPropType=SimpleVisualProperties  GraphicDiffuseColor=smiData.Solid(5).color  GraphicSpecularColor=[0.5 0.5 0.5 1.0]  GraphicAmbientColor=[0.15 0.15 0.15 1.0]  GraphicEmissiveColor=[0.0 0.0 0.0 1.0]  GraphicShininess=75  GraphicOpacity=smiData.Solid(5).opacity  GeometryShape=FromFile  RectangleSize=[1 1]  RectangleSizeUnits=m  BrickDimensions=[1 1 1]  BrickDimensionUnits=m  CylinderRadius=1  CylinderRadiusUnits=m  CylinderLength=1  CylinderLengthUnits=m  SphereRadius=1  SphereRadiusUnits=m  EllipsoidRadii=[1 1 1]  EllipsoidRadiiUnits=m  ExtrusionCrossSection=[1 1; -1 1; -1 -1; 1 -1]  ExtrusionCrossSectionUnits=m  ExtrusionLength=1  ExtrusionLengthUnits=m  PolygonNumSides=3  PolygonOuterRadius=1  PolygonOuterRadiusUnits=m  ExtGeomFileType=STEP  ExtGeomFileName=link2_Default_sldprt.STEP  ExtGeomFileUnits=m  RevolutionCrossSection=[1 1; 1 -1; 2 -1; 2 1]  RevolutionCrossSectionUnits=m  RevolutionExtent=Full  RevolutionAngle=180  RevolutionAngleUnits=deg
  Transform : sm_lib/Frames and Transforms/Rigid Transform  TranslationMethod=Cartesian  TranslationStandardOffset=0  TranslationLengthUnit=m  TranslationStandardAxis=+Z  TranslationCartesianOffset=smiData.RigidTransform(2).translation  TranslationROffset=0  TranslationROffsetUnits=m  TranslationZOffset=0  TranslationZOffsetUnits=m  TranslationThetaOffset=0  TranslationThetaOffsetUnits=deg  RotationMethod=ArbitraryAxis  RotationAngleUnits=rad  RotationStandardAxis=+Z  RotationAngle=smiData.RigidTransform(2).angle  RotationArbitraryAxis=smiData.RigidTransform(2).axis  FollAlignAxisA=+X  BaseAlignAxisA=+Y  FollAlignAxisB=+Y  BaseAlignAxisB=+Z  RotationSequenceAxes=FollowerAxes  RotationSequence=XYX  RotationSequenceAngles=[0 0 0]  RotationSequenceAnglesUnits=deg  RotationMatrix=[1 0 0; 0 1 0; 0 0 1]
  Transform1 : sm_lib/Frames and Transforms/Rigid Transform  TranslationMethod=Cartesian  TranslationStandardOffset=0  TranslationLengthUnit=m  TranslationStandardAxis=+Z  TranslationCartesianOffset=smiData.RigidTransform(5).translation  TranslationROffset=0  TranslationROffsetUnits=m  TranslationZOffset=0  TranslationZOffsetUnits=m  TranslationThetaOffset=0  TranslationThetaOffsetUnits=deg  RotationMethod=ArbitraryAxis  RotationAngleUnits=rad  RotationStandardAxis=+Z  RotationAngle=smiData.RigidTransform(5).angle  RotationArbitraryAxis=smiData.RigidTransform(5).axis  FollAlignAxisA=+X  BaseAlignAxisA=+Y  FollAlignAxisB=+Y  BaseAlignAxisB=+Z  RotationSequenceAxes=FollowerAxes  RotationSequence=XYX  RotationSequenceAngles=[0 0 0]  RotationSequenceAnglesUnits=deg  RotationMatrix=[1 0 0; 0 1 0; 0 0 1]
  F : PMIOPort  Side=Left
  F1 : PMIOPort  Port=2  Side=Right
  connections:
  Solid/RConn1 -- ReferenceFrame/RConn1 -- Transform/LConn1 -- Transform1/LConn1
  Transform/RConn1 -- F/RConn1
  Transform1/RConn1 -- F1/RConn1

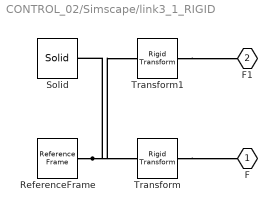
== system CONTROL_02/Simscape/link3_1_RIGID ==
  ReferenceFrame : sm_lib/Frames and Transforms/Reference Frame
  Solid : sm_lib/Body Elements/Solid  InertiaType=Custom  Mass=smiData.Solid(3).mass  MassUnits=kg  CenterOfMass=smiData.Solid(3).CoM  CenterOfMassUnits=m  MomentsOfInertia=smiData.Solid(3).MoI  MomentsOfInertiaUnits=kg*m^2  ProductsOfInertia=smiData.Solid(3).PoI  ProductsOfInertiaUnits=kg*m^2  BasedOnType=Density  Density=1000  DensityUnits=kg/m^3  DoExposeReferenceFrame=on  SerializedFrames=<Frames/>  GraphicType=FromGeometry  MarkerShape=Sphere  MarkerSize=10  GraphicVisPropType=SimpleVisualProperties  GraphicDiffuseColor=smiData.Solid(3).color  GraphicSpecularColor=[0.5 0.5 0.5 1.0]  GraphicAmbientColor=[0.15 0.15 0.15 1.0]  GraphicEmissiveColor=[0.0 0.0 0.0 1.0]  GraphicShininess=75  GraphicOpacity=smiData.Solid(3).opacity  GeometryShape=FromFile  RectangleSize=[1 1]  RectangleSizeUnits=m  BrickDimensions=[1 1 1]  BrickDimensionUnits=m  CylinderRadius=1  CylinderRadiusUnits=m  CylinderLength=1  CylinderLengthUnits=m  SphereRadius=1  SphereRadiusUnits=m  EllipsoidRadii=[1 1 1]  EllipsoidRadiiUnits=m  ExtrusionCrossSection=[1 1; -1 1; -1 -1; 1 -1]  ExtrusionCrossSectionUnits=m  ExtrusionLength=1  ExtrusionLengthUnits=m  PolygonNumSides=3  PolygonOuterRadius=1  PolygonOuterRadiusUnits=m  ExtGeomFileType=STEP  ExtGeomFileName=link3_Default_sldprt.STEP  ExtGeomFileUnits=m  RevolutionCrossSection=[1 1; 1 -1; 2 -1; 2 1]  RevolutionCrossSectionUnits=m  RevolutionExtent=Full  RevolutionAngle=180  RevolutionAngleUnits=deg
  Transform : sm_lib/Frames and Transforms/Rigid Transform  TranslationMethod=Cartesian  TranslationStandardOffset=0  TranslationLengthUnit=m  TranslationStandardAxis=+Z  TranslationCartesianOffset=smiData.RigidTransform(6).translation  TranslationROffset=0  TranslationROffsetUnits=m  TranslationZOffset=0  TranslationZOffsetUnits=m  TranslationThetaOffset=0  TranslationThetaOffsetUnits=deg  RotationMethod=ArbitraryAxis  RotationAngleUnits=rad  RotationStandardAxis=+Z  RotationAngle=smiData.RigidTransform(6).angle  RotationArbitraryAxis=smiData.RigidTransform(6).axis  FollAlignAxisA=+X  BaseAlignAxisA=+Y  FollAlignAxisB=+Y  BaseAlignAxisB=+Z  RotationSequenceAxes=FollowerAxes  RotationSequence=XYX  RotationSequenceAngles=[0 0 0]  RotationSequenceAnglesUnits=deg  RotationMatrix=[1 0 0; 0 1 0; 0 0 1]
  Transform1 : sm_lib/Frames and Transforms/Rigid Transform  TranslationMethod=Cartesian  TranslationStandardOffset=0  TranslationLengthUnit=m  TranslationStandardAxis=+Z  TranslationCartesianOffset=smiData.RigidTransform(7).translation  TranslationROffset=0  TranslationROffsetUnits=m  TranslationZOffset=0  TranslationZOffsetUnits=m  TranslationThetaOffset=0  TranslationThetaOffsetUnits=deg  RotationMethod=ArbitraryAxis  RotationAngleUnits=rad  RotationStandardAxis=+Z  RotationAngle=smiData.RigidTransform(7).angle  RotationArbitraryAxis=smiData.RigidTransform(7).axis  FollAlignAxisA=+X  BaseAlignAxisA=+Y  FollAlignAxisB=+Y  BaseAlignAxisB=+Z  RotationSequenceAxes=FollowerAxes  RotationSequence=XYX  RotationSequenceAngles=[0 0 0]  RotationSequenceAnglesUnits=deg  RotationMatrix=[1 0 0; 0 1 0; 0 0 1]
  F : PMIOPort  Side=Left
  F1 : PMIOPort  Port=2  Side=Right
  connections:
  Solid/RConn1 -- ReferenceFrame/RConn1 -- Transform/LConn1 -- Transform1/LConn1
  Transform/RConn1 -- F/RConn1
  Transform1/RConn1 -- F1/RConn1

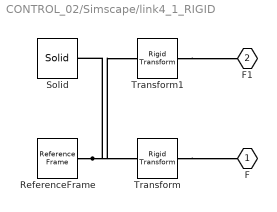
== system CONTROL_02/Simscape/link4_1_RIGID ==
  ReferenceFrame : sm_lib/Frames and Transforms/Reference Frame
  Solid : sm_lib/Body Elements/Solid  InertiaType=Custom  Mass=smiData.Solid(4).mass  MassUnits=kg  CenterOfMass=smiData.Solid(4).CoM  CenterOfMassUnits=m  MomentsOfInertia=smiData.Solid(4).MoI  MomentsOfInertiaUnits=kg*m^2  ProductsOfInertia=smiData.Solid(4).PoI  ProductsOfInertiaUnits=kg*m^2  BasedOnType=Density  Density=1000  DensityUnits=kg/m^3  DoExposeReferenceFrame=on  SerializedFrames=<Frames/>  GraphicType=FromGeometry  MarkerShape=Sphere  MarkerSize=10  GraphicVisPropType=SimpleVisualProperties  GraphicDiffuseColor=smiData.Solid(4).color  GraphicSpecularColor=[0.5 0.5 0.5 1.0]  GraphicAmbientColor=[0.15 0.15 0.15 1.0]  GraphicEmissiveColor=[0.0 0.0 0.0 1.0]  GraphicShininess=75  GraphicOpacity=smiData.Solid(4).opacity  GeometryShape=FromFile  RectangleSize=[1 1]  RectangleSizeUnits=m  BrickDimensions=[1 1 1]  BrickDimensionUnits=m  CylinderRadius=1  CylinderRadiusUnits=m  CylinderLength=1  CylinderLengthUnits=m  SphereRadius=1  SphereRadiusUnits=m  EllipsoidRadii=[1 1 1]  EllipsoidRadiiUnits=m  ExtrusionCrossSection=[1 1; -1 1; -1 -1; 1 -1]  ExtrusionCrossSectionUnits=m  ExtrusionLength=1  ExtrusionLengthUnits=m  PolygonNumSides=3  PolygonOuterRadius=1  PolygonOuterRadiusUnits=m  ExtGeomFileType=STEP  ExtGeomFileName=link4_Default_sldprt.STEP  ExtGeomFileUnits=m  RevolutionCrossSection=[1 1; 1 -1; 2 -1; 2 1]  RevolutionCrossSectionUnits=m  RevolutionExtent=Full  RevolutionAngle=180  RevolutionAngleUnits=deg
  Transform : sm_lib/Frames and Transforms/Rigid Transform  TranslationMethod=Cartesian  TranslationStandardOffset=0  TranslationLengthUnit=m  TranslationStandardAxis=+Z  TranslationCartesianOffset=smiData.RigidTransform(8).translation  TranslationROffset=0  TranslationROffsetUnits=m  TranslationZOffset=0  TranslationZOffsetUnits=m  TranslationThetaOffset=0  TranslationThetaOffsetUnits=deg  RotationMethod=ArbitraryAxis  RotationAngleUnits=rad  RotationStandardAxis=+Z  RotationAngle=smiData.RigidTransform(8).angle  RotationArbitraryAxis=smiData.RigidTransform(8).axis  FollAlignAxisA=+X  BaseAlignAxisA=+Y  FollAlignAxisB=+Y  BaseAlignAxisB=+Z  RotationSequenceAxes=FollowerAxes  RotationSequence=XYX  RotationSequenceAngles=[0 0 0]  RotationSequenceAnglesUnits=deg  RotationMatrix=[1 0 0; 0 1 0; 0 0 1]
  Transform1 : sm_lib/Frames and Transforms/Rigid Transform  TranslationMethod=Cartesian  TranslationStandardOffset=0  TranslationLengthUnit=m  TranslationStandardAxis=+Z  TranslationCartesianOffset=smiData.RigidTransform(9).translation  TranslationROffset=0  TranslationROffsetUnits=m  TranslationZOffset=0  TranslationZOffsetUnits=m  TranslationThetaOffset=0  TranslationThetaOffsetUnits=deg  RotationMethod=ArbitraryAxis  RotationAngleUnits=rad  RotationStandardAxis=+Z  RotationAngle=smiData.RigidTransform(9).angle  RotationArbitraryAxis=smiData.RigidTransform(9).axis  FollAlignAxisA=+X  BaseAlignAxisA=+Y  FollAlignAxisB=+Y  BaseAlignAxisB=+Z  RotationSequenceAxes=FollowerAxes  RotationSequence=XYX  RotationSequenceAngles=[0 0 0]  RotationSequenceAnglesUnits=deg  RotationMatrix=[1 0 0; 0 1 0; 0 0 1]
  F : PMIOPort  Side=Left
  F1 : PMIOPort  Port=2  Side=Right
  connections:
  Solid/RConn1 -- ReferenceFrame/RConn1 -- Transform/LConn1 -- Transform1/LConn1
  Transform/RConn1 -- F/RConn1
  Transform1/RConn1 -- F1/RConn1

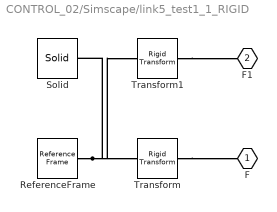
== system CONTROL_02/Simscape/link5_test1_1_RIGID ==
  ReferenceFrame : sm_lib/Frames and Transforms/Reference Frame
  Solid : sm_lib/Body Elements/Solid  InertiaType=Custom  Mass=smiData.Solid(6).mass  MassUnits=kg  CenterOfMass=smiData.Solid(6).CoM  CenterOfMassUnits=m  MomentsOfInertia=smiData.Solid(6).MoI  MomentsOfInertiaUnits=kg*m^2  ProductsOfInertia=smiData.Solid(6).PoI  ProductsOfInertiaUnits=kg*m^2  BasedOnType=Density  Density=1000  DensityUnits=kg/m^3  DoExposeReferenceFrame=on  SerializedFrames=<Frames/>  GraphicType=FromGeometry  MarkerShape=Sphere  MarkerSize=10  GraphicVisPropType=SimpleVisualProperties  GraphicDiffuseColor=smiData.Solid(6).color  GraphicSpecularColor=[0.5 0.5 0.5 1.0]  GraphicAmbientColor=[0.15 0.15 0.15 1.0]  GraphicEmissiveColor=[0.0 0.0 0.0 1.0]  GraphicShininess=75  GraphicOpacity=smiData.Solid(6).opacity  GeometryShape=FromFile  RectangleSize=[1 1]  RectangleSizeUnits=m  BrickDimensions=[1 1 1]  BrickDimensionUnits=m  CylinderRadius=1  CylinderRadiusUnits=m  CylinderLength=1  CylinderLengthUnits=m  SphereRadius=1  SphereRadiusUnits=m  EllipsoidRadii=[1 1 1]  EllipsoidRadiiUnits=m  ExtrusionCrossSection=[1 1; -1 1; -1 -1; 1 -1]  ExtrusionCrossSectionUnits=m  ExtrusionLength=1  ExtrusionLengthUnits=m  PolygonNumSides=3  PolygonOuterRadius=1  PolygonOuterRadiusUnits=m  ExtGeomFileType=STEP  ExtGeomFileName=link5_test1_Default_sldprt.STEP  ExtGeomFileUnits=m  RevolutionCrossSection=[1 1; 1 -1; 2 -1; 2 1]  RevolutionCrossSectionUnits=m  RevolutionExtent=Full  RevolutionAngle=180  RevolutionAngleUnits=deg
  Transform : sm_lib/Frames and Transforms/Rigid Transform  TranslationMethod=Cartesian  TranslationStandardOffset=0  TranslationLengthUnit=m  TranslationStandardAxis=+Z  TranslationCartesianOffset=smiData.RigidTransform(10).translation  TranslationROffset=0  TranslationROffsetUnits=m  TranslationZOffset=0  TranslationZOffsetUnits=m  TranslationThetaOffset=0  TranslationThetaOffsetUnits=deg  RotationMethod=ArbitraryAxis  RotationAngleUnits=rad  RotationStandardAxis=+Z  RotationAngle=smiData.RigidTransform(10).angle  RotationArbitraryAxis=smiData.RigidTransform(10).axis  FollAlignAxisA=+X  BaseAlignAxisA=+Y  FollAlignAxisB=+Y  BaseAlignAxisB=+Z  RotationSequenceAxes=FollowerAxes  RotationSequence=XYX  RotationSequenceAngles=[0 0 0]  RotationSequenceAnglesUnits=deg  RotationMatrix=[1 0 0; 0 1 0; 0 0 1]
  Transform1 : sm_lib/Frames and Transforms/Rigid Transform  TranslationMethod=Cartesian  TranslationStandardOffset=0  TranslationLengthUnit=m  TranslationStandardAxis=+Z  TranslationCartesianOffset=smiData.RigidTransform(11).translation  TranslationROffset=0  TranslationROffsetUnits=m  TranslationZOffset=0  TranslationZOffsetUnits=m  TranslationThetaOffset=0  TranslationThetaOffsetUnits=deg  RotationMethod=ArbitraryAxis  RotationAngleUnits=rad  RotationStandardAxis=+Z  RotationAngle=smiData.RigidTransform(11).angle  RotationArbitraryAxis=smiData.RigidTransform(11).axis  FollAlignAxisA=+X  BaseAlignAxisA=+Y  FollAlignAxisB=+Y  BaseAlignAxisB=+Z  RotationSequenceAxes=FollowerAxes  RotationSequence=XYX  RotationSequenceAngles=[0 0 0]  RotationSequenceAnglesUnits=deg  RotationMatrix=[1 0 0; 0 1 0; 0 0 1]
  F : PMIOPort  Side=Left
  F1 : PMIOPort  Port=2  Side=Right
  connections:
  Solid/RConn1 -- ReferenceFrame/RConn1 -- Transform/LConn1 -- Transform1/LConn1
  Transform/RConn1 -- F/RConn1
  Transform1/RConn1 -- F1/RConn1

== system CONTROL_02/Simscape/link5_test2_2_RIGID ==
  ReferenceFrame : sm_lib/Frames and Transforms/Reference Frame
  Solid : sm_lib/Body Elements/Solid  InertiaType=Custom  Mass=smiData.Solid(7).mass  MassUnits=kg  CenterOfMass=smiData.Solid(7).CoM  CenterOfMassUnits=m  MomentsOfInertia=smiData.Solid(7).MoI  MomentsOfInertiaUnits=kg*m^2  ProductsOfInertia=smiData.Solid(7).PoI  ProductsOfInertiaUnits=kg*m^2  BasedOnType=Density  Density=1000  DensityUnits=kg/m^3  DoExposeReferenceFrame=on  SerializedFrames=<Frames/>  GraphicType=FromGeometry  MarkerShape=Sphere  MarkerSize=10  GraphicVisPropType=SimpleVisualProperties  GraphicDiffuseColor=smiData.Solid(7).color  GraphicSpecularColor=[0.5 0.5 0.5 1.0]  GraphicAmbientColor=[0.15 0.15 0.15 1.0]  GraphicEmissiveColor=[0.0 0.0 0.0 1.0]  GraphicShininess=75  GraphicOpacity=smiData.Solid(7).opacity  GeometryShape=FromFile  RectangleSize=[1 1]  RectangleSizeUnits=m  BrickDimensions=[1 1 1]  BrickDimensionUnits=m  CylinderRadius=1  CylinderRadiusUnits=m  CylinderLength=1  CylinderLengthUnits=m  SphereRadius=1  SphereRadiusUnits=m  EllipsoidRadii=[1 1 1]  EllipsoidRadiiUnits=m  ExtrusionCrossSection=[1 1; -1 1; -1 -1; 1 -1]  ExtrusionCrossSectionUnits=m  ExtrusionLength=1  ExtrusionLengthUnits=m  PolygonNumSides=3  PolygonOuterRadius=1  PolygonOuterRadiusUnits=m  ExtGeomFileType=STEP  ExtGeomFileName=link5_test2_Default_sldprt.STEP  ExtGeomFileUnits=m  RevolutionCrossSection=[1 1; 1 -1; 2 -1; 2 1]  RevolutionCrossSectionUnits=m  RevolutionExtent=Full  RevolutionAngle=180  RevolutionAngleUnits=deg
  Transform : sm_lib/Frames and Transforms/Rigid Transform  TranslationMethod=Cartesian  TranslationStandardOffset=0  TranslationLengthUnit=m  TranslationStandardAxis=+Z  TranslationCartesianOffset=smiData.RigidTransform(12).translation  TranslationROffset=0  TranslationROffsetUnits=m  TranslationZOffset=0  TranslationZOffsetUnits=m  TranslationThetaOffset=0  TranslationThetaOffsetUnits=deg  RotationMethod=ArbitraryAxis  RotationAngleUnits=rad  RotationStandardAxis=+Z  RotationAngle=smiData.RigidTransform(12).angle  RotationArbitraryAxis=smiData.RigidTransform(12).axis  FollAlignAxisA=+X  BaseAlignAxisA=+Y  FollAlignAxisB=+Y  BaseAlignAxisB=+Z  RotationSequenceAxes=FollowerAxes  RotationSequence=XYX  RotationSequenceAngles=[0 0 0]  RotationSequenceAnglesUnits=deg  RotationMatrix=[1 0 0; 0 1 0; 0 0 1]
  F : PMIOPort  Side=Left
  connections:
  Solid/RConn1 -- ReferenceFrame/RConn1 -- Transform/LConn1
  Transform/RConn1 -- F/RConn1

== matlab function CONTROL_02/6DOF Manipulator/Dynamics ==
  data: de input; t input; Fe input; M input; ddthe output; C input; G input; J input; dt output; ex output
function [ddthe,dt,ex] = DYN_6DOF(de,t,Fe,M,C,G,J)
%%
% Fv: viscous friction 2
% Fc: Coulomb friction 2
% Fe: External Force
Fc = 0.01*diag([1,1,1,1,1,1]);
% Fv = diag([5,5,5,0.5,0.1,0.05]);
% Fv = 0.14*diag([2,4,4,1,1,1]);
Fv = 0.01*diag([1,1,1,1,1,1]);
% dt: Model error + External disturbance
dt = Fc*sign(de) + Fv*de + J.'*Fe;
ex = J.'*Fe;
%%
ddthe = inv(M)*(t - C*de - G - dt);
